simulink model "chart_model"  (Simulink 8.9)
settings: Solver=FixedStepDiscrete  StartTime=0.0  StopTime=10.0  FixedStep=0.1  RelTol=1e-3  EnableMultiTasking=on
values from neighbouring files (symbols this model uses):
  Ts = 1    [lab_script.m]
libraries: dspsrcs4 x1
settings Model: Creator=Ира  LastModifiedBy=Ира
settings SolverCC: AutoInsertRateTranBlk=on
settings DataIOCC: SaveFormat=Dataset  SignalLoggingSaveFormat=Dataset
settings DebuggingCC: UnderspecifiedInitializationDetection=Simplified  MergeDetectMultiDrivingBlocksExec=error  FcnCallInpInsideContextMsg=error  AllowSymbolicDim=off  StateNameClashWarn=none
settings HardwareCC: ProdBitPerPointer=64  ProdBitPerSizeT=64  ProdBitPerPtrDiffT=64  ProdLargestAtomicFloat=Float  ProdIntDivRoundTo=Zero  ProdEndianess=LittleEndian  ProdWordSize=64  ProdHWDeviceType=Intel->x86-64 (Windows64)
settings ModelReferenceCC: PropagateSignalLabelsOutOfModel=on
settings GRTTargetCC: CombineOutputUpdateFcns=on  GRTInterface=off
settings ConfigComp: CovShowResultsExplorer=off  CovSFcnEnable=off

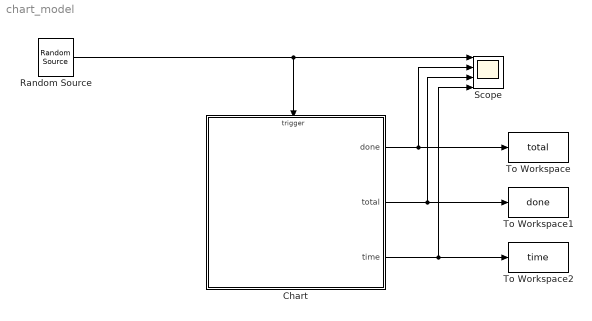
== system chart_model ==
  Chart : Stateflow chart  TreatAsAtomicUnit=on
  Random Source : dspsrcs4/Random Source  SrcType=Gaussian  NormMethod=Sum of uniform values  CltLength=12  MinVal=0  MaxVal=1  MeanVal=Li  VarVal=1  RepMode=Not repeatable  rawSeed=1  IsInherit=off  SampMode=Discrete  SampTime=Ts  SampFrame=1  DataType=Double  OutComplex=Real  OutputFrames=off
  Scope : Scope  NumInputPorts=4
  To Workspace : ToWorkspace  VariableName=total  SampleTime=Ts
  To Workspace1 : ToWorkspace  VariableName=done  SampleTime=Ts
  To Workspace2 : ToWorkspace  VariableName=time  SampleTime=Ts
  wires:
  Chart/1(done) -> To Workspace/1, Scope/2
  Chart/2(total) -> Scope/3, To Workspace1/1
  Chart/3(time) -> Scope/4, To Workspace2/1
  Random Source/1 -> Chart/Trigger, Scope/1

== stateflow chart Chart ==
  state Q1 [parallel]
    settings: executionOrder=2
    state ProcessQ1 [parallel]
      settings: executionOrder=1
      state free/
      state busy/
        entry:bt1=ml('prand(1/Lo)');
        to1=t;
        during: time = time + 1;
        exit: done = done + 1;
      (default) -> Q1.ProcessQ1.free
      Q1.ProcessQ1.free -> Q1.ProcessQ1.busy : setrequest
      (junction 29) -> Q1.ProcessQ1.free [order 2]
      (junction 29) -> Q1.ProcessQ1.busy [order 1] : [nq1>0]
          | {send(getrequest, QueueQ1);}
      Q1.ProcessQ1.busy -> (junction 29) : [t-to1>=bt1]
    state QueueQ1 [parallel]
      settings: executionOrder=2
      state empty/
      state stored/
        on setrequest: nq1 = nq1 + 1;
        on getrequest: nq1 = nq1 - 1;
        during:time=time+nq1;
      state full/
        during:time=time+nq1;
      Q1.QueueQ1.empty -> Q1.QueueQ1.stored : setrequest/
          | {nq1 = nq1 + 1;}
      (default) -> Q1.QueueQ1.empty
      Q1.QueueQ1.stored -> Q1.QueueQ1.empty [order 2] : [nq1==0]
      Q1.QueueQ1.full -> Q1.QueueQ1.stored : getrequest/
          | {nq1 = nq1 - 1;}
      Q1.QueueQ1.stored -> Q1.QueueQ1.full [order 1] : [nq1==ml.nqm1]
  state Q2 [parallel]
    settings: executionOrder=3
    state ProcessQ2 [parallel]
      settings: executionOrder=1
      state free/
      state busy/
        entry:bt2=ml('prand(1/Lo)');
        to2=t;
        during: time = time + 1;
        exit: done = done + 1;
      Q2.ProcessQ2.free -> Q2.ProcessQ2.busy : setrequest
      (default) -> Q2.ProcessQ2.free
      (junction 40) -> Q2.ProcessQ2.free [order 2]
      (junction 40) -> Q2.ProcessQ2.busy [order 1] : [nq2>0]
          | {send(getrequest, QueueQ2);}
      Q2.ProcessQ2.busy -> (junction 40) : [t-to2>=bt2]
    state QueueQ2 [parallel]
      settings: executionOrder=2
      state full/
        during:time=time+nq2;
      state stored/
        on setrequest: nq2 = nq2 + 1;
        on getrequest: nq2 = nq2 - 1;
        during:time=time+nq2;
      state empty/
      (default) -> Q2.QueueQ2.empty
      Q2.QueueQ2.empty -> Q2.QueueQ2.stored : setrequest/
          | {nq2 = nq2 + 1;}
      Q2.QueueQ2.stored -> Q2.QueueQ2.empty [order 2] : [nq2==0]
      Q2.QueueQ2.full -> Q2.QueueQ2.stored : getrequest/
          | {nq2 = nq2 - 1;}
      Q2.QueueQ2.stored -> Q2.QueueQ2.full [order 1] : [nq2==ml.nqm2]
  state Active [parallel]
    settings: executionOrder=1
    state main/
    (default) -> main
    main -> (junction 21) : request/
        | {total = total + 1;}
    (junction 21) -> main [order 5]
    (junction 21) -> main [order 1] : [in(ProcessQ1.free)]
        | {send(setrequest, ProcessQ1)}
    (junction 21) -> main [order 4] : [in(~QueueQ2.full)]
        | {send(setrequest, QueueQ2)}
    (junction 21) -> main [order 3] : [in(~QueueQ1.full)]
        | {send(setrequest, QueueQ1)}
    (junction 21) -> main [order 2] : [in(ProcessQ2.free)]
        | {send(setrequest, ProcessQ2)}
  data: bt1 local double; to1 local double; nq1 local double; nq2 local double; to2 local double; bt2 local double; done output double; total output double; time output double
  data bt1 settings: description=% length of queue
  data to1 settings: description=% length of queue
  data nq1 settings: description=% length of queue
  data nq2 settings: description=% length of queue
  data to2 settings: description=% length of queue
  data bt2 settings: description=% length of queue
  data done settings: description=% length of queue
  data total settings: description=% length of queue
  data time settings: description=% length of queue
  events: request input RISING_EDGE_EVENT; setrequest local FUNCTION_CALL_EVENT; getrequest local FUNCTION_CALL_EVENT
